simulink model "Vergleich_L1"  (Simulink 7.8)
settings: Solver=ode45  StartTime=0.0  StopTime=30  MaxStep=1e-4  RelTol=1e-3
values from neighbouring files (symbols this model uses):
  A = [0,1;-0.4,-0.5]    [Vergleich_MRAC_L1.m]
  Am = [0,1;-2,-2]    [Vergleich_MRAC_L1.m]
  b = [0;1]    [Vergleich_MRAC_L1.m]
  c = [1,0]    [Vergleich_MRAC_L1.m]
  cm = [1,0]    [Vergleich_MRAC_L1.m]
  Gamma1 = 100000    [Vergleich_MRAC_L1.m]
  kg = -1/(c*inv(Am)*b)    [Vergleich_MRAC_L1.m]
  km = [1.6,1.5]    [Vergleich_MRAC_L1.m]
  omega = 40    [Vergleich_MRAC_L1.m]    (also in lambda_plot.m = i)
  Pb = P*b    [Vergleich_MRAC_L1.m]
  theta = [1,-1]    [Vergleich_MRAC_L1.m]
libraries: vrlib x2, simulink x1
settings Model: Creator=Markus  LastModifiedBy=Markus

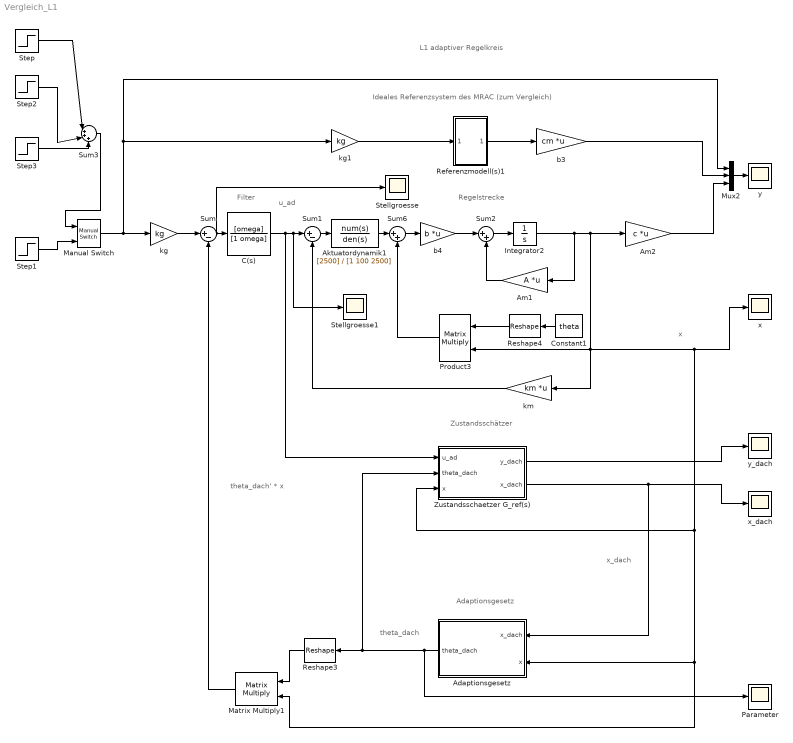
== system Vergleich_L1 ==
  note: Regelstrecke
  note: Zustandsschätzer
  note: Adaptionsgesetz
  note: theta_dach' * x
  note: L1 adaptiver Regelkreis
  note: x_dach
  note: x
  note: theta_dach
  note: Filter
  note: u_ad
  note: Ideales Referenzsystem des MRAC (zum Vergleich)
  Adaptionsgesetz : Subsystem
  Aktuatordynamik1 : TransferFcn  Numerator=[2500]  Denominator=[1 100 2500]
  Am1 : Gain  Gain=A  Multiplication=Matrix(K*u)
  Am2 : Gain  Gain=c  Multiplication=Matrix(K*u)
  C(s) : TransferFcn  Numerator=[omega]  Denominator=[1 omega]
  Constant1 : Constant  Value=theta
  Integrator2 : Integrator
  Manual Switch : simulink/Signal Routing/Manual Switch  sw=1  action=0  varsize=off
  Matrix Multiply1 : Product  Multiplication=Matrix(*)
  Mux2 : Mux  Inputs=3
  Parameter : Scope
      settings: TimeRange=0.01659605551497442  YMin=0.3  YMax=1.05  SaveName=simout
  Product3 : Product  Multiplication=Matrix(*)  RndMeth=Zero
  Referenzmodell(s)1 : Subsystem
  Reshape3 : Reshape  OutputDimensionality=Row vector (2-D)
  Reshape4 : Reshape  OutputDimensionality=Row vector (2-D)
  Stellgroesse : Scope
      settings: TimeRange=0.01659605551497442  YMin=12.0476  YMax=12.0494  SaveName=simout1
  Stellgroesse1 : Scope
      settings: TimeRange=0.01659605551497442  YMin=-2  YMax=7.5  SaveName=simout2
  Step : Step  SampleTime=0
  Step1 : Step  SampleTime=0
  Step2 : Step  Time=11  SampleTime=0
  Step3 : Step  Time=21  After=2  SampleTime=0
  Sum : Sum  Inputs=|+-
  Sum1 : Sum  Inputs=|+-
  Sum2 : Sum  Inputs=|++
  Sum3 : Sum  Inputs=|+++
  Sum6 : Sum  Inputs=|++
  Zustandsschaetzer G_ref(s) : Subsystem
  b3 : Gain  Gain=cm  Multiplication=Matrix(K*u)
  b4 : Gain  Gain=b  Multiplication=Matrix(K*u)
  kg : Gain  Gain=kg
  kg1 : Gain  Gain=kg
  km : Gain  Gain=km  Multiplication=Matrix(K*u)
  x : Scope
      settings: YMin=0  YMax=110  SaveName=ScopeData3
  x_dach : Scope
      settings: YMin=0  YMax=2.5  SaveName=ScopeData4
  y : Scope
      settings: TimeRange=6.7353579175705  YMin=3.6  YMax=4.1  SaveName=Sim_data4  DataFormat=Array
  y_dach : Scope
      settings: YMin=0  YMax=35
  wires:
  kg/1 -> Sum/1
  Sum/1 -> C(s)/1, Stellgroesse/1
  Matrix Multiply1/1 -> Sum/2
  Reshape3/1 -> Matrix Multiply1/1
  Adaptionsgesetz/1(theta_dach) -> Reshape3/1, Zustandsschaetzer G_ref(s)/2(theta_dach), Parameter/1
  Zustandsschaetzer G_ref(s)/2(x_dach) -> Adaptionsgesetz/1(x_dach), x_dach/1
  b3/1 -> Mux2/2
  Mux2/1 -> y/1
  C(s)/1 -> Zustandsschaetzer G_ref(s)/1(u_ad), Sum1/1, Stellgroesse1/1
  Referenzmodell(s)1/1(Out1) -> b3/1
  Integrator2/1 -> Am1/1, Product3/2, Am2/1, Matrix Multiply1/2, Adaptionsgesetz/2(x), Zustandsschaetzer G_ref(s)/3(x), x/1, km/1
  Sum2/1 -> Integrator2/1
  b4/1 -> Sum2/1
  Constant1/1 -> Reshape4/1
  Reshape4/1 -> Product3/1
  Am1/1 -> Sum2/2
  Sum6/1 -> b4/1
  Manual Switch/1 -> kg/1, Mux2/1, kg1/1
  Step1/1 -> Manual Switch/2
  Am2/1 -> Mux2/3
  Zustandsschaetzer G_ref(s)/1(y_dach) -> y_dach/1
  km/1 -> Sum1/2
  kg1/1 -> Referenzmodell(s)1/1(In1)
  Product3/1 -> Sum6/2
  Step/1 -> Sum3/1
  Step2/1 -> Sum3/2
  Step3/1 -> Sum3/3
  Sum3/1 -> Manual Switch/1
  Sum1/1 -> Aktuatordynamik1/1
  Aktuatordynamik1/1 -> Sum6/1

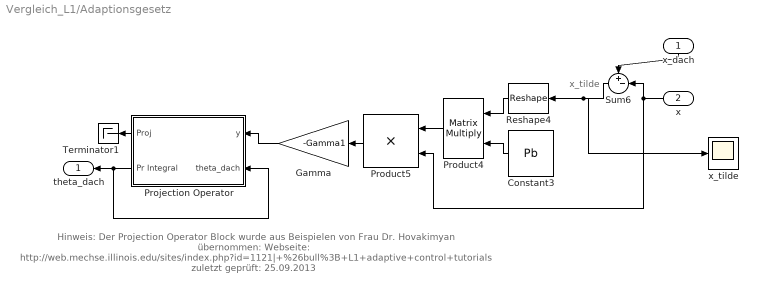
== system Vergleich_L1/Adaptionsgesetz ==
  note: x_tilde
  note: Hinweis: Der Projection Operator Block wurde aus Beispielen von Frau Dr. Hovakimyan übernommen:
      | Webseite: http://web.mechse.illinois.edu/sites/index.php?id=1121|+%26bull%3B+L1+adaptive+control+tutorials
      | zuletzt geprüft: 25.09.2013
  x_dach : Inport
  x : Inport  Port=2
  Constant3 : Constant  Value=Pb
  Gamma : Gain  Gain=-Gamma1
  Product4 : Product  Multiplication=Matrix(*)  RndMeth=Zero
  Product5 : Product  RndMeth=Zero
  Projection Operator : Subsystem  mask{EpsilonTheta=0.03, Prmax=2, Pr0=0}
      mask prompts: EpsilonTheta "Epsilon"; Prmax "Bound (radius of the ball)"; Pr0 "Initialization of integral"
      mask help:
      | Computes projection of the signal and safely integrate it.
      | Works both for scalar and vector signals.
      | It considers the parameter set as a ball at the origin with setted radius.
      mask init:
      | Thetamax = Prmax / sqrt(EpsilonTheta+1);
  Reshape4 : Reshape  OutputDimensionality=Row vector (2-D)
  Sum6 : Sum  Inputs=+-|
  Terminator1 : Terminator
  x_tilde : Scope
      settings: YMin=0  YMax=35  SaveName=ScopeData2
  theta_dach : Outport
  wires:
  Sum6/1 -> Reshape4/1, x_tilde/1
  Reshape4/1 -> Product4/1
  Constant3/1 -> Product4/2
  Product4/1 -> Product5/1
  Product5/1 -> Gamma/1
  Gamma/1 -> Projection Operator/1(y)
  Projection Operator/2(Pr Integral) -> theta_dach/1, Projection Operator/2(theta_dach)
  Projection Operator/1(Proj) -> Terminator1/1
  x_dach/1 -> Sum6/1
  x/1 -> Sum6/2, Product5/2

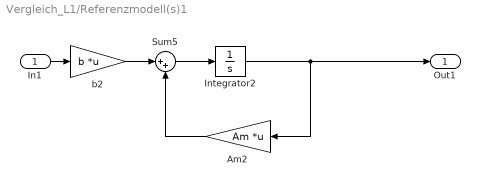
== system Vergleich_L1/Referenzmodell(s)1 ==
  In1 : Inport  PortDimensions=[1,1]
  Am2 : Gain  Gain=Am  Multiplication=Matrix(K*u)
  Integrator2 : Integrator
  Sum5 : Sum  Inputs=|++
  b2 : Gain  Gain=b  Multiplication=Matrix(K*u)
  Out1 : Outport
  wires:
  Integrator2/1 -> Am2/1, Out1/1
  Sum5/1 -> Integrator2/1
  b2/1 -> Sum5/1
  Am2/1 -> Sum5/2
  In1/1 -> b2/1

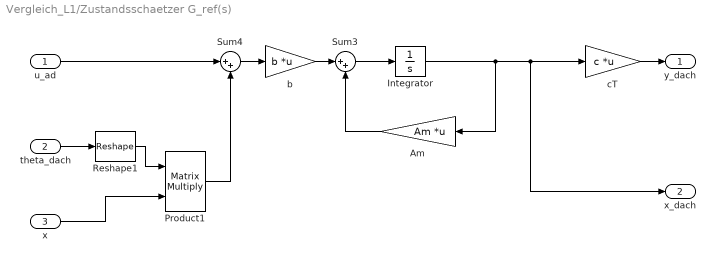
== system Vergleich_L1/Zustandsschaetzer G_ref(s) ==
  u_ad : Inport
  theta_dach : Inport  Port=2
  x : Inport  Port=3
  Am : Gain  Gain=Am  Multiplication=Matrix(K*u)
  Integrator : Integrator
  Product1 : Product  Multiplication=Matrix(*)  RndMeth=Zero
  Reshape1 : Reshape  OutputDimensionality=Row vector (2-D)
  Sum3 : Sum  Inputs=|++
  Sum4 : Sum  Inputs=|++
  b : Gain  Gain=b  Multiplication=Matrix(K*u)
  cT : Gain  Gain=c  Multiplication=Matrix(K*u)
  y_dach : Outport
  x_dach : Outport  Port=2
  wires:
  Integrator/1 -> Am/1, cT/1, x_dach/1
  Sum3/1 -> Integrator/1
  b/1 -> Sum3/1
  Am/1 -> Sum3/2
  Sum4/1 -> b/1
  u_ad/1 -> Sum4/1
  cT/1 -> y_dach/1
  theta_dach/1 -> Reshape1/1
  Reshape1/1 -> Product1/1
  x/1 -> Product1/2
  Product1/1 -> Sum4/2

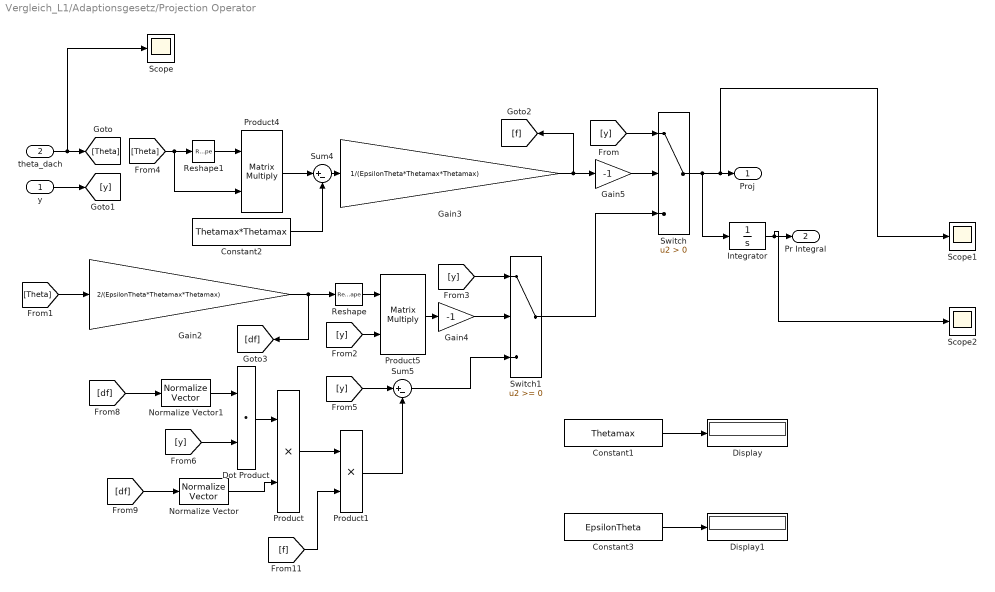
== system Vergleich_L1/Adaptionsgesetz/Projection Operator ==
  y : Inport
  theta_dach : Inport  Port=2
  Constant1 : Constant  Value=Thetamax  VectorParams1D=off
  Constant2 : Constant  Value=Thetamax*Thetamax
  Constant3 : Constant  Value=EpsilonTheta  VectorParams1D=off
  Display : Display
  Display1 : Display
  Dot Product : DotProduct  InputSameDT=on  OutDataTypeStr=Inherit: Inherit via internal rule
  Gain2 : Gain  Gain=2/(EpsilonTheta*Thetamax*Thetamax)
  Gain3 : Gain  Gain=1/(EpsilonTheta*Thetamax*Thetamax)
  Gain4 : Gain  Gain=-1
  Gain5 : Gain  Gain=-1
  Integrator : Integrator  InitialCondition=Pr0  LimitOutput=on  UpperSaturationLimit=Prmax  LowerSaturationLimit=-Prmax
  Normalize Vector : vrlib/Utilities/Normalize Vector  maxzero=0
  Normalize Vector1 : vrlib/Utilities/Normalize Vector  maxzero=0
  Product : Product  RndMeth=Zero
  Product1 : Product  RndMeth=Zero
  Product4 : Product  Multiplication=Matrix(*)  RndMeth=Zero
  Product5 : Product  Multiplication=Matrix(*)  RndMeth=Zero
  Reshape : Reshape  OutputDimensionality=Row vector (2-D)
  Reshape1 : Reshape  OutputDimensionality=Row vector (2-D)
  Scope : Scope
      settings: YMin=-6  YMax=9  SaveName=ScopeData8
  Scope1 : Scope
      settings: YMin=-150000  YMax=150000  SaveName=ScopeData9
  Scope2 : Scope
      settings: YMin=-6  YMax=9  SaveName=ScopeData10
  Sum4 : Sum  Inputs=|+-
  Sum5 : Sum  Inputs=|+-
  Switch : Switch  Criteria=u2 > Threshold
  Switch1 : Switch
  Proj : Outport
  Pr Integral : Outport  Port=2
  wires:
  Gain5/1 -> Switch/2
  Sum5/1 -> Switch1/3
  [y] -> Sum5/1
  theta_dach/1 -> [Theta], Scope/1
  y/1 -> [y]
  Switch/1 -> Integrator/1, Proj/1, Scope1/1
  Switch1/1 -> Switch/3
  [Theta] -> Gain2/1
  [y] -> Switch1/1
  Gain4/1 -> Switch1/2
  Product5/1 -> Gain4/1
  [y] -> Product5/2
  [y] -> Switch/1
  Gain3/1 -> [f], Gain5/1
  Sum4/1 -> Gain3/1
  Constant2/1 -> Sum4/2
  [Theta] -> Reshape1/1, Product4/2
  Gain2/1 -> Reshape/1, [df]
  Reshape/1 -> Product5/1
  Reshape1/1 -> Product4/1
  [df] -> Normalize Vector1/1
  [df] -> Normalize Vector/1
  Normalize Vector1/1 -> Dot Product/1
  [y] -> Dot Product/2
  Dot Product/1 -> Product/1
  Normalize Vector/1 -> Product/2
  Product/1 -> Product1/1
  [f] -> Product1/2
  Product1/1 -> Sum5/2
  Integrator/1 -> Pr Integral/1, Scope2/1
  Constant1/1 -> Display/1
  Constant3/1 -> Display1/1
  Product4/1 -> Sum4/1
